simulink model "model3"  (R2024a)
settings: Solver=VariableStepAuto  StartTime=0.0  StopTime=10.0  RelTol=1e-3
settings Model: Creator=TAU  LastModifiedBy=TAU

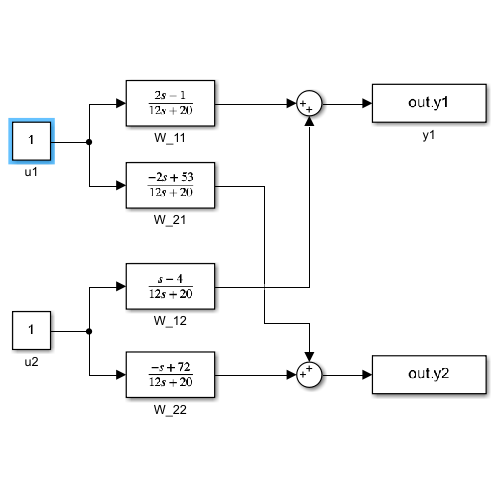
[thumbnail: Simulink's stored preview of the top-level diagram]
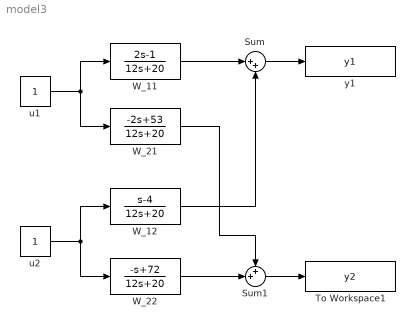
== system model3 ==
  Sum : Sum  Inputs=|++
  Sum1 : Sum  Inputs=++|
  To Workspace1 : ToWorkspace  VariableName=y2  SaveFormat=Timeseries  SampleTime=-1
  W_11 : TransferFcn  Numerator=[2 -1]  Denominator=[12 20]
  W_12 : TransferFcn  Numerator=[1 -4]  Denominator=[12 20]
  W_21 : TransferFcn  Numerator=[-2 53]  Denominator=[12 20]
  W_22 : TransferFcn  Numerator=[-1 72]  Denominator=[12 20]
  u1 : Constant
  u2 : Constant
  y1 : ToWorkspace  VariableName=y1  SaveFormat=Timeseries  SampleTime=-1
  wires:
  u2/1 -> W_22/1, W_12/1
  u1/1 -> W_21/1, W_11/1
  W_12/1 -> Sum/2
  W_11/1 -> Sum/1
  W_22/1 -> Sum1/2
  W_21/1 -> Sum1/1
  Sum/1 -> y1/1
  Sum1/1 -> To Workspace1/1
